simulink model "simli"  (R2023b)
settings: Solver=VariableStepAuto  StartTime=0.0  StopTime=10  RelTol=1e-3
undefined symbols (not defined in the file or in its folder): c_f, C_hv_km, Cagg, Cbase1v, Cbase_hv, Cbase_mv, delta_vsc_0, G_dc_denom, G_dc_num, H_gen, H_vsm, i_d_vsc, i_q_vsc, Ibase_hv, Ibase_mv, k_d_vsm, k_p_p_vsm, k_p_q_vsm, k_vc, ki, ki_q, kp, L_comp, l_f, l_grid, L_hv_km, l_t_ehvhv, l_t_hvmv, l_t_mvlv, Lagg, Lbase_hv, Lbase_mv, length_export, M_gr_denom, M_gr_num, mppt_gain, omega_nom, omega_WTR_0, omega_WTR_n, P_aero_0, P_meas, phase_shift_test_state, phase_shifts, pie_export, Q_meas, r_cf, r_f, r_grid, R_hv_km, r_sys, r_t_ehvhv, r_t_hvmv, r_t_mvlv, Ragg, Rd, rocof_slope, Rocof_test_state, T_dc_denom, T_dc_num, Tdelay ... (+18)
libraries: slpidlib x9, spsFirstOrderFilterLib x1, simulink x1, spsSampleandHoldLib x1, spspowerguiLib x1
(part 3 of 3)

== system simli/Subsystem/WT transformer  ==
  note: Network
  note: VIRTUAL RESITANCE
  Vpcc_DQ : Inport
  "VsDQ " : Inport  Port=2
  omega_ref : Inport  Port=3
  1 : Gain  Gain=inv_Lsource
  2 : Gain  Gain=Rsource
  3 : Gain  Gain=Rsource
  4 : Gain  Gain=inv_Lsource
  7 : Gain  Gain=Lsource
  Demux1 : Demux  Outputs=2
  Demux2 : Demux  Outputs=2
  Id : Scope
  Iline_D_int : Integrator  UpperSaturationLimit=50  LowerSaturationLimit=-1000
  Iline_Q_int : Integrator  UpperSaturationLimit=50  LowerSaturationLimit=-1000
  Iq : Scope
  Mux1 : Mux  Inputs=2
  Mux4 : Mux  Inputs=2
  Product1 : Product
  Product2 : Product
  Sum1 : Sum  Inputs=|+---
  Sum8 : Sum  Inputs=|+-+-
  Iline_DQ : Outport  VectorParamsAs1DForOutWhenUnconnected=off
  wires:
  7/1 -> [wL]
  [Vpcc_Q] -> Sum1/1
  [Vpcc_D] -> Sum8/1
  Demux2/1 -> Mux4/1, [Vpcc_D]
  Demux2/2 -> Mux4/2, [Vpcc_Q]
  Sum1/1 -> 4/1
  1/1 -> Iline_D_int/1
  Iline_D_int/1 -> Product1/2, Id/1, 2/1, Mux1/1
  Iline_Q_int/1 -> Mux1/2, Iq/1, Product2/2, 3/1
  Sum8/1 -> 1/1
  2/1 -> Sum8/4
  Product2/1 -> Sum8/3
  3/1 -> Sum1/4
  4/1 -> Iline_Q_int/1
  Product1/1 -> Sum1/3
  [wL] -> Product1/1, Product2/1
  Demux1/1 -> Sum8/2
  Demux1/2 -> Sum1/2
  "VsDQ "/1 -> Demux1/1
  Vpcc_DQ/1 -> Demux2/1
  Mux1/1 -> Iline_DQ/1
  omega_ref/1 -> 7/1

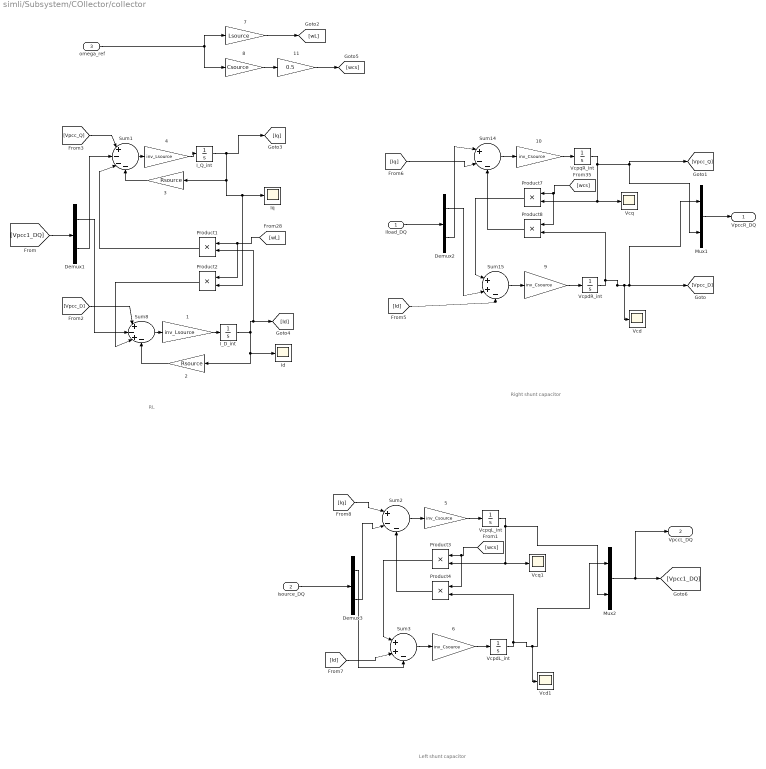
== system simli/Subsystem/COllector/collector ==
  note: RL
  note: Right shunt capacitor
  note: Left shunt capacitor
  Iload_DQ : Inport
  "Isource_DQ " : Inport  Port=2
  omega_ref : Inport  Port=3
  1 : Gain  Gain=inv_Lsource
  {5..6,9..10} (4 alike) : Gain  Gain=inv_Csource
  11 : Gain  Gain=0.5
  2 : Gain  Gain=Rsource
  3 : Gain  Gain=Rsource
  4 : Gain  Gain=inv_Lsource
  7 : Gain  Gain=Lsource
  8 : Gain  Gain=Csource
  Demux1 : Demux  Outputs=2
  Demux2 : Demux  Outputs=2
  Demux3 : Demux  Outputs=2
  I_D_int : Integrator  UpperSaturationLimit=50  LowerSaturationLimit=-1000
  I_Q_int : Integrator  UpperSaturationLimit=50  LowerSaturationLimit=-1000
  Id : Scope
  Iq : Scope
  Mux1 : Mux  Inputs=2
  Mux2 : Mux  Inputs=2
  Product{1..4,7..8} (6 alike) : Product
  Sum1 : Sum  Inputs=|+---
  Sum14 : Sum  Inputs=|+--
  Sum15 : Sum  Inputs=|++-
  Sum2 : Sum  Inputs=|+--
  Sum3 : Sum  Inputs=|++-
  Sum8 : Sum  Inputs=|+-+-
  Vcd : Scope
  Vcd1 : Scope
  VcpdL_int : Integrator  UpperSaturationLimit=50  LowerSaturationLimit=-1000
  VcpdR_int : Integrator  UpperSaturationLimit=50  LowerSaturationLimit=-1000
  VcpqL_int : Integrator  UpperSaturationLimit=50  LowerSaturationLimit=-1000
  VcpqR_int : Integrator  UpperSaturationLimit=50  LowerSaturationLimit=-1000
  Vcq : Scope
  Vcq1 : Scope
  VpccR_DQ : Outport  VectorParamsAs1DForOutWhenUnconnected=off
  VpccL_DQ : Outport  Port=2  VectorParamsAs1DForOutWhenUnconnected=off
  wires:
  Iload_DQ/1 -> Demux2/1
  Demux2/2 -> Sum14/1
  Demux2/1 -> Sum15/2
  [wL] -> Product2/1, Product1/1
  Product1/1 -> Sum1/3
  4/1 -> I_Q_int/1
  3/1 -> Sum1/4
  Product2/1 -> Sum8/3
  2/1 -> Sum8/4
  Sum8/1 -> 1/1
  I_Q_int/1 -> 3/1, Product2/2, Iq/1, [Iq]
  I_D_int/1 -> 2/1, Id/1, Product1/2, [Id]
  1/1 -> I_D_int/1
  Sum1/1 -> 4/1
  [Vpcc_D] -> Sum8/1
  [Vpcc_Q] -> Sum1/1
  omega_ref/1 -> 8/1, 7/1
  7/1 -> [wL]
  9/1 -> VcpdR_int/1
  Sum14/1 -> 10/1
  [wcs] -> Product8/1, Product7/1
  [Id] -> Sum15/3
  VcpqR_int/1 -> Mux1/2, [Vpcc_Q], Product7/2, Vcq/1
  Product7/1 -> Sum15/1
  [Iq] -> Sum14/2
  10/1 -> VcpqR_int/1
  Sum15/1 -> 9/1
  Product8/1 -> Sum14/3
  8/1 -> 11/1
  VcpdR_int/1 -> Product8/2, Mux1/1, [Vpcc_D], Vcd/1
  Mux1/1 -> VpccR_DQ/1
  Demux1/1 -> Sum8/2
  Demux1/2 -> Sum1/2
  [Vpcc1_DQ] -> Demux1/1
  VcpdL_int/1 -> Vcd1/1, Mux2/1, Product4/2
  Product4/1 -> Sum2/3
  Sum3/1 -> 6/1
  5/1 -> VcpqL_int/1
  Demux3/2 -> Sum2/2
  Product3/1 -> Sum3/1
  VcpqL_int/1 -> Vcq1/1, Product3/2, Mux2/2
  [wcs] -> Product3/1, Product4/1
  Sum2/1 -> 5/1
  6/1 -> VcpdL_int/1
  "Isource_DQ "/1 -> Demux3/1
  Demux3/1 -> Sum3/3
  [Id] -> Sum3/2
  [Iq] -> Sum2/1
  Mux2/1 -> VpccL_DQ/1, [Vpcc1_DQ]
  11/1 -> [wcs]

== system simli/Subsystem/HVAC CABLE 10 PI SEGMENTS 1/RC sys1 ==
  note: Left shunt capacitor
  note: shunt capacitor
  Iload_DQ : Inport
  "Isource_DQ " : Inport  Port=2
  omega_ref : Inport  Port=3
  1 : Gain  Gain=Rd
  10 : Gain  Gain=inv_Csource
  2 : Gain  Gain=Rd
  8 : Gain  Gain=Csource
  9 : Gain  Gain=inv_Csource
  Demux2 : Demux  Outputs=2
  Demux3 : Demux  Outputs=2
  Display1 : Display
  Display6 : Display
  Mux1 : Mux  Inputs=2
  Mux2 : Mux  Inputs=2
  Product7 : Product
  Product8 : Product
  Sum1 : Sum  Inputs=|++
  Sum14 : Sum  Inputs=|+--
  Sum15 : Sum  Inputs=|++-
  Sum2 : Sum  Inputs=|++
  Sum3 : Sum  Inputs=|+-
  Sum4 : Sum  Inputs=|+-
  Vcd : Scope
  VcpdR_int : Integrator  InitialCondition=VD0  UpperSaturationLimit=50  LowerSaturationLimit=-1000
  VcpqR_int : Integrator  InitialCondition=VQ0  UpperSaturationLimit=50  LowerSaturationLimit=-1000
  Vcq : Scope
  VpccR_DQ : Outport  VectorParamsAs1DForOutWhenUnconnected=off
  wires:
  8/1 -> [wcs], Display1/1
  Mux1/1 -> VpccR_DQ/1
  Product8/1 -> Sum14/3
  Sum15/1 -> 9/1
  10/1 -> VcpqR_int/1
  Product7/1 -> Sum15/1
  VcpqR_int/1 -> Mux2/1, Sum2/1, Product7/2, Vcq/1
  [wcs] -> Product7/1, Product8/1
  Sum14/1 -> 10/1
  9/1 -> VcpdR_int/1
  omega_ref/1 -> 8/1
  Demux2/1 -> Sum4/1, Sum15/2
  Demux2/2 -> Sum3/1, Sum14/1
  Iload_DQ/1 -> Demux2/1
  "Isource_DQ "/1 -> Demux3/1
  Demux3/2 -> Sum3/2, Sum14/2
  Demux3/1 -> Sum4/2, Sum15/3
  VcpdR_int/1 -> Mux2/2, Product8/2, Sum1/1
  Sum1/1 -> Mux1/1
  Sum2/1 -> Mux1/2
  1/1 -> Sum2/2
  2/1 -> Sum1/2
  Mux2/1 -> Display6/1
  Sum3/1 -> 1/1
  Sum4/1 -> 2/1

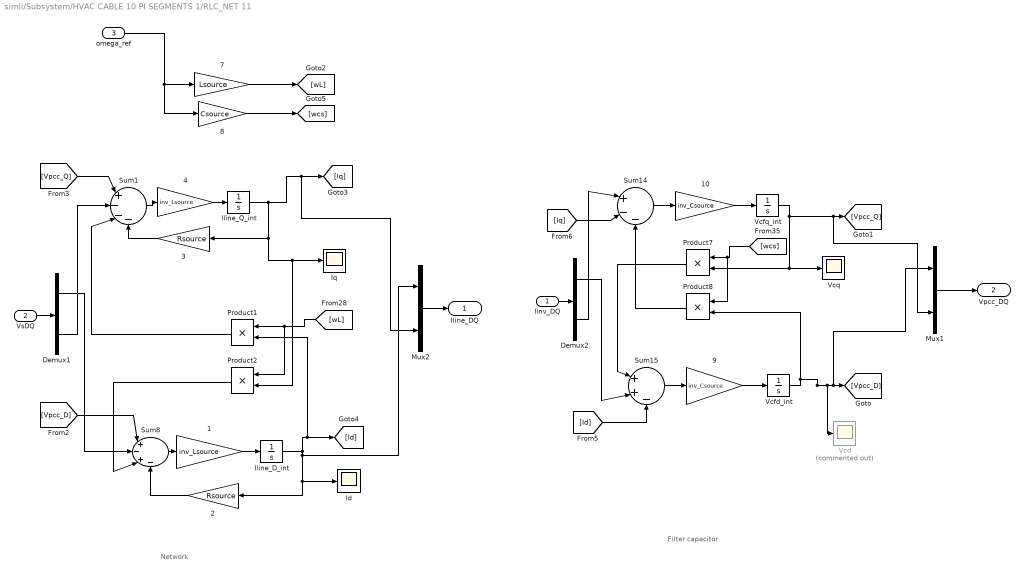
== system simli/Subsystem/HVAC CABLE 10 PI SEGMENTS 1/RLC_NET 11 ==
  note: Network
  note: Filter capacitor
  Iinv_DQ : Inport
  "VsDQ " : Inport  Port=2
  omega_ref : Inport  Port=3
  1 : Gain  Gain=inv_Lsource
  10 : Gain  Gain=inv_Csource
  2 : Gain  Gain=Rsource
  3 : Gain  Gain=Rsource
  4 : Gain  Gain=inv_Lsource
  7 : Gain  Gain=Lsource
  8 : Gain  Gain=Csource
  9 : Gain  Gain=inv_Csource
  Demux1 : Demux  Outputs=2
  Demux2 : Demux  Outputs=2
  Id : Scope
  Iline_D_int : Integrator  UpperSaturationLimit=50  LowerSaturationLimit=-1000
  Iline_Q_int : Integrator  UpperSaturationLimit=50  LowerSaturationLimit=-1000
  Iq : Scope
  Mux1 : Mux  Inputs=2
  Mux2 : Mux  Inputs=2
  Product{1..2,7..8} (4 alike) : Product
  Sum1 : Sum  Inputs=|+---
  Sum14 : Sum  Inputs=|+--
  Sum15 : Sum  Inputs=|++-
  Sum8 : Sum  Inputs=|+-+-
  Vcd : Scope  Commented=on
  Vcfd_int : Integrator  UpperSaturationLimit=50  LowerSaturationLimit=-1000
  Vcfq_int : Integrator  UpperSaturationLimit=50  LowerSaturationLimit=-1000
  Vcq : Scope
  Iline_DQ : Outport  VectorParamsAs1DForOutWhenUnconnected=off
  Vpcc_DQ : Outport  Port=2  VectorParamsAs1DForOutWhenUnconnected=off
  wires:
  Mux2/1 -> Iline_DQ/1
  Iinv_DQ/1 -> Demux2/1
  Demux2/2 -> Sum14/1
  Demux2/1 -> Sum15/2
  [wL] -> Product2/1, Product1/1
  Product1/1 -> Sum1/3
  4/1 -> Iline_Q_int/1
  3/1 -> Sum1/4
  Product2/1 -> Sum8/3
  2/1 -> Sum8/4
  Sum8/1 -> 1/1
  Iline_Q_int/1 -> 3/1, Product2/2, Iq/1, [Iq], Mux2/2
  Iline_D_int/1 -> Mux2/1, 2/1, Id/1, Product1/2, [Id]
  1/1 -> Iline_D_int/1
  Sum1/1 -> 4/1
  [Vpcc_D] -> Sum8/1
  [Vpcc_Q] -> Sum1/1
  omega_ref/1 -> 8/1, 7/1
  7/1 -> [wL]
  9/1 -> Vcfd_int/1
  Sum14/1 -> 10/1
  [wcs] -> Product8/1, Product7/1
  [Id] -> Sum15/3
  Vcfq_int/1 -> Mux1/2, [Vpcc_Q], Product7/2, Vcq/1
  Product7/1 -> Sum15/1
  [Iq] -> Sum14/2
  10/1 -> Vcfq_int/1
  Sum15/1 -> 9/1
  Product8/1 -> Sum14/3
  8/1 -> [wcs]
  Vcfd_int/1 -> Product8/2, Mux1/1, [Vpcc_D], Vcd/1
  Mux1/1 -> Vpcc_DQ/1
  Demux1/1 -> Sum8/2
  Demux1/2 -> Sum1/2
  "VsDQ "/1 -> Demux1/1

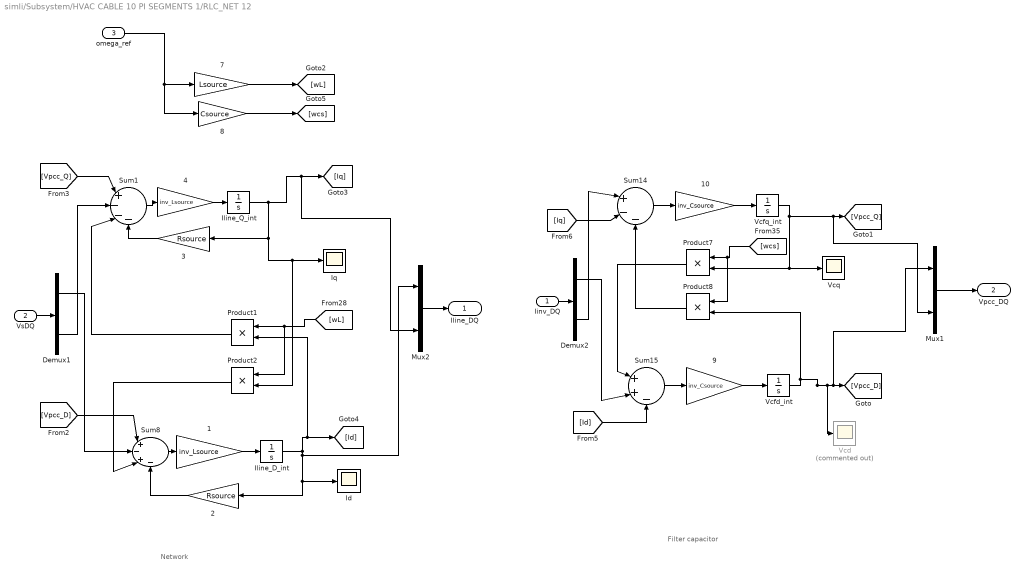
== system simli/Subsystem/HVAC CABLE 10 PI SEGMENTS 1/RLC_NET 12 ==
  note: Filter capacitor
  note: Network
  Iinv_DQ : Inport
  "VsDQ " : Inport  Port=2
  omega_ref : Inport  Port=3
  1 : Gain  Gain=inv_Lsource
  10 : Gain  Gain=inv_Csource
  2 : Gain  Gain=Rsource
  3 : Gain  Gain=Rsource
  4 : Gain  Gain=inv_Lsource
  7 : Gain  Gain=Lsource
  8 : Gain  Gain=Csource
  9 : Gain  Gain=inv_Csource
  Demux1 : Demux  Outputs=2
  Demux2 : Demux  Outputs=2
  Id : Scope
  Iline_D_int : Integrator  UpperSaturationLimit=50  LowerSaturationLimit=-1000
  Iline_Q_int : Integrator  UpperSaturationLimit=50  LowerSaturationLimit=-1000
  Iq : Scope
  Mux1 : Mux  Inputs=2
  Mux2 : Mux  Inputs=2
  Product{1..2,7..8} (4 alike) : Product
  Sum1 : Sum  Inputs=|+---
  Sum14 : Sum  Inputs=|+--
  Sum15 : Sum  Inputs=|++-
  Sum8 : Sum  Inputs=|+-+-
  Vcd : Scope  Commented=on
  Vcfd_int : Integrator  UpperSaturationLimit=50  LowerSaturationLimit=-1000
  Vcfq_int : Integrator  UpperSaturationLimit=50  LowerSaturationLimit=-1000
  Vcq : Scope
  Iline_DQ : Outport  VectorParamsAs1DForOutWhenUnconnected=off
  Vpcc_DQ : Outport  Port=2  VectorParamsAs1DForOutWhenUnconnected=off
  wires:
  "VsDQ "/1 -> Demux1/1
  Demux1/2 -> Sum1/2
  Demux1/1 -> Sum8/2
  Mux1/1 -> Vpcc_DQ/1
  Vcfd_int/1 -> Vcd/1, [Vpcc_D], Mux1/1, Product8/2
  8/1 -> [wcs]
  Product8/1 -> Sum14/3
  Sum15/1 -> 9/1
  10/1 -> Vcfq_int/1
  [Iq] -> Sum14/2
  Product7/1 -> Sum15/1
  Vcfq_int/1 -> Vcq/1, Product7/2, [Vpcc_Q], Mux1/2
  [Id] -> Sum15/3
  [wcs] -> Product7/1, Product8/1
  Sum14/1 -> 10/1
  9/1 -> Vcfd_int/1
  7/1 -> [wL]
  omega_ref/1 -> 7/1, 8/1
  [Vpcc_Q] -> Sum1/1
  [Vpcc_D] -> Sum8/1
  Sum1/1 -> 4/1
  1/1 -> Iline_D_int/1
  Iline_D_int/1 -> [Id], Product1/2, Id/1, 2/1, Mux2/1
  Iline_Q_int/1 -> Mux2/2, [Iq], Iq/1, Product2/2, 3/1
  Sum8/1 -> 1/1
  2/1 -> Sum8/4
  Product2/1 -> Sum8/3
  3/1 -> Sum1/4
  4/1 -> Iline_Q_int/1
  Product1/1 -> Sum1/3
  [wL] -> Product1/1, Product2/1
  Demux2/1 -> Sum15/2
  Demux2/2 -> Sum14/1
  Iinv_DQ/1 -> Demux2/1
  Mux2/1 -> Iline_DQ/1

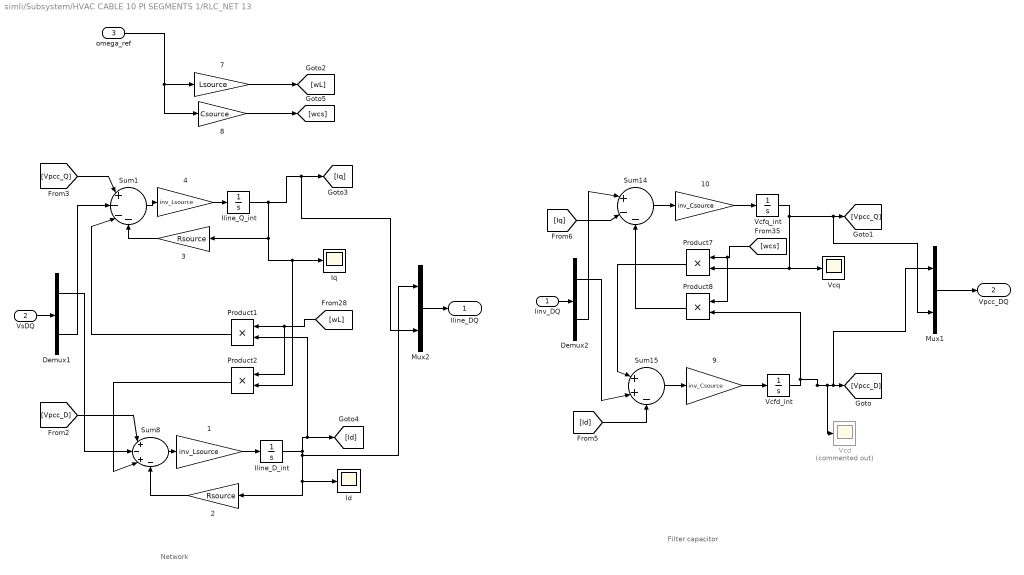
== system simli/Subsystem/HVAC CABLE 10 PI SEGMENTS 1/RLC_NET 13 ==
  note: Filter capacitor
  note: Network
  Iinv_DQ : Inport
  "VsDQ " : Inport  Port=2
  omega_ref : Inport  Port=3
  1 : Gain  Gain=inv_Lsource
  10 : Gain  Gain=inv_Csource
  2 : Gain  Gain=Rsource
  3 : Gain  Gain=Rsource
  4 : Gain  Gain=inv_Lsource
  7 : Gain  Gain=Lsource
  8 : Gain  Gain=Csource
  9 : Gain  Gain=inv_Csource
  Demux1 : Demux  Outputs=2
  Demux2 : Demux  Outputs=2
  Id : Scope
  Iline_D_int : Integrator  UpperSaturationLimit=50  LowerSaturationLimit=-1000
  Iline_Q_int : Integrator  UpperSaturationLimit=50  LowerSaturationLimit=-1000
  Iq : Scope
  Mux1 : Mux  Inputs=2
  Mux2 : Mux  Inputs=2
  Product{1..2,7..8} (4 alike) : Product
  Sum1 : Sum  Inputs=|+---
  Sum14 : Sum  Inputs=|+--
  Sum15 : Sum  Inputs=|++-
  Sum8 : Sum  Inputs=|+-+-
  Vcd : Scope  Commented=on
  Vcfd_int : Integrator  UpperSaturationLimit=50  LowerSaturationLimit=-1000
  Vcfq_int : Integrator  UpperSaturationLimit=50  LowerSaturationLimit=-1000
  Vcq : Scope
  Iline_DQ : Outport  VectorParamsAs1DForOutWhenUnconnected=off
  Vpcc_DQ : Outport  Port=2  VectorParamsAs1DForOutWhenUnconnected=off
  wires:
  "VsDQ "/1 -> Demux1/1
  Demux1/2 -> Sum1/2
  Demux1/1 -> Sum8/2
  Mux1/1 -> Vpcc_DQ/1
  Vcfd_int/1 -> Vcd/1, [Vpcc_D], Mux1/1, Product8/2
  8/1 -> [wcs]
  Product8/1 -> Sum14/3
  Sum15/1 -> 9/1
  10/1 -> Vcfq_int/1
  [Iq] -> Sum14/2
  Product7/1 -> Sum15/1
  Vcfq_int/1 -> Vcq/1, Product7/2, [Vpcc_Q], Mux1/2
  [Id] -> Sum15/3
  [wcs] -> Product7/1, Product8/1
  Sum14/1 -> 10/1
  9/1 -> Vcfd_int/1
  7/1 -> [wL]
  omega_ref/1 -> 7/1, 8/1
  [Vpcc_Q] -> Sum1/1
  [Vpcc_D] -> Sum8/1
  Sum1/1 -> 4/1
  1/1 -> Iline_D_int/1
  Iline_D_int/1 -> [Id], Product1/2, Id/1, 2/1, Mux2/1
  Iline_Q_int/1 -> Mux2/2, [Iq], Iq/1, Product2/2, 3/1
  Sum8/1 -> 1/1
  2/1 -> Sum8/4
  Product2/1 -> Sum8/3
  3/1 -> Sum1/4
  4/1 -> Iline_Q_int/1
  Product1/1 -> Sum1/3
  [wL] -> Product1/1, Product2/1
  Demux2/1 -> Sum15/2
  Demux2/2 -> Sum14/1
  Iinv_DQ/1 -> Demux2/1
  Mux2/1 -> Iline_DQ/1

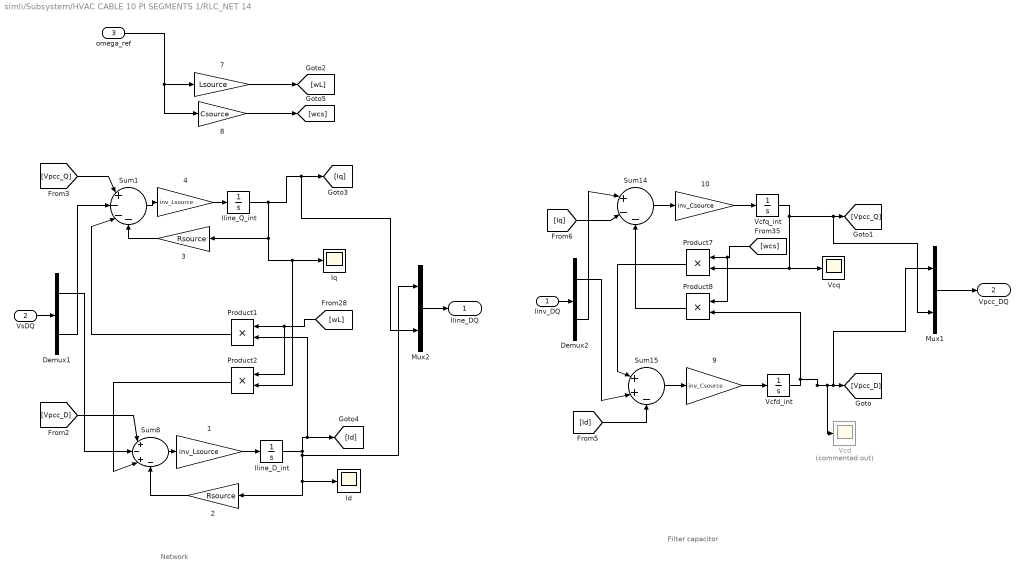
== system simli/Subsystem/HVAC CABLE 10 PI SEGMENTS 1/RLC_NET 14 ==
  note: Network
  note: Filter capacitor
  Iinv_DQ : Inport
  "VsDQ " : Inport  Port=2
  omega_ref : Inport  Port=3
  1 : Gain  Gain=inv_Lsource
  10 : Gain  Gain=inv_Csource
  2 : Gain  Gain=Rsource
  3 : Gain  Gain=Rsource
  4 : Gain  Gain=inv_Lsource
  7 : Gain  Gain=Lsource
  8 : Gain  Gain=Csource
  9 : Gain  Gain=inv_Csource
  Demux1 : Demux  Outputs=2
  Demux2 : Demux  Outputs=2
  Id : Scope
  Iline_D_int : Integrator  UpperSaturationLimit=50  LowerSaturationLimit=-1000
  Iline_Q_int : Integrator  UpperSaturationLimit=50  LowerSaturationLimit=-1000
  Iq : Scope
  Mux1 : Mux  Inputs=2
  Mux2 : Mux  Inputs=2
  Product{1..2,7..8} (4 alike) : Product
  Sum1 : Sum  Inputs=|+---
  Sum14 : Sum  Inputs=|+--
  Sum15 : Sum  Inputs=|++-
  Sum8 : Sum  Inputs=|+-+-
  Vcd : Scope  Commented=on
  Vcfd_int : Integrator  UpperSaturationLimit=50  LowerSaturationLimit=-1000
  Vcfq_int : Integrator  UpperSaturationLimit=50  LowerSaturationLimit=-1000
  Vcq : Scope
  Iline_DQ : Outport  VectorParamsAs1DForOutWhenUnconnected=off
  Vpcc_DQ : Outport  Port=2  VectorParamsAs1DForOutWhenUnconnected=off
  wires:
  Mux2/1 -> Iline_DQ/1
  Iinv_DQ/1 -> Demux2/1
  Demux2/2 -> Sum14/1
  Demux2/1 -> Sum15/2
  [wL] -> Product2/1, Product1/1
  Product1/1 -> Sum1/3
  4/1 -> Iline_Q_int/1
  3/1 -> Sum1/4
  Product2/1 -> Sum8/3
  2/1 -> Sum8/4
  Sum8/1 -> 1/1
  Iline_Q_int/1 -> 3/1, Product2/2, Iq/1, [Iq], Mux2/2
  Iline_D_int/1 -> Mux2/1, 2/1, Id/1, Product1/2, [Id]
  1/1 -> Iline_D_int/1
  Sum1/1 -> 4/1
  [Vpcc_D] -> Sum8/1
  [Vpcc_Q] -> Sum1/1
  omega_ref/1 -> 8/1, 7/1
  7/1 -> [wL]
  9/1 -> Vcfd_int/1
  Sum14/1 -> 10/1
  [wcs] -> Product8/1, Product7/1
  [Id] -> Sum15/3
  Vcfq_int/1 -> Mux1/2, [Vpcc_Q], Product7/2, Vcq/1
  Product7/1 -> Sum15/1
  [Iq] -> Sum14/2
  10/1 -> Vcfq_int/1
  Sum15/1 -> 9/1
  Product8/1 -> Sum14/3
  8/1 -> [wcs]
  Vcfd_int/1 -> Product8/2, Mux1/1, [Vpcc_D], Vcd/1
  Mux1/1 -> Vpcc_DQ/1
  Demux1/1 -> Sum8/2
  Demux1/2 -> Sum1/2
  "VsDQ "/1 -> Demux1/1

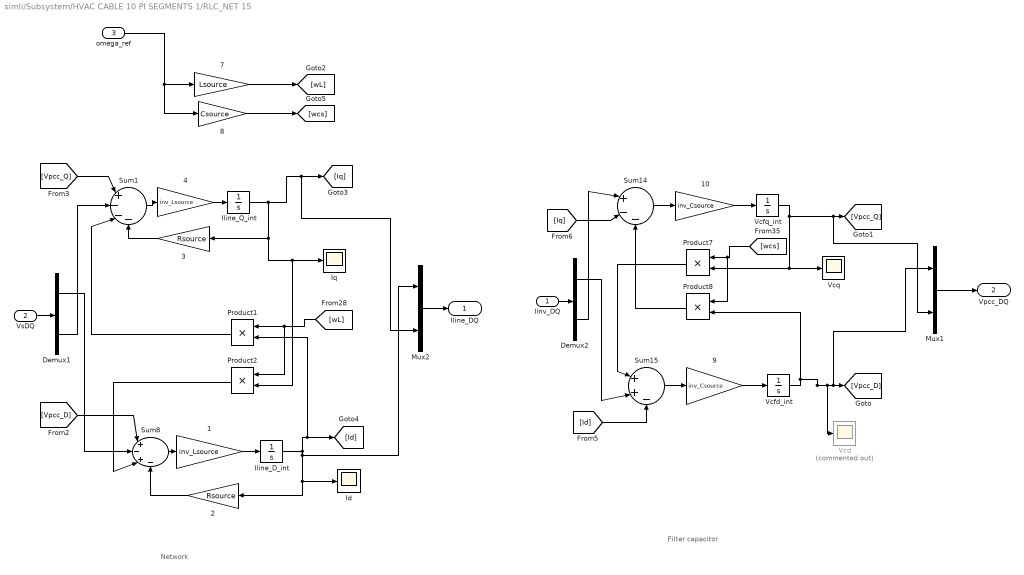
== system simli/Subsystem/HVAC CABLE 10 PI SEGMENTS 1/RLC_NET 15 ==
  note: Filter capacitor
  note: Network
  Iinv_DQ : Inport
  "VsDQ " : Inport  Port=2
  omega_ref : Inport  Port=3
  1 : Gain  Gain=inv_Lsource
  10 : Gain  Gain=inv_Csource
  2 : Gain  Gain=Rsource
  3 : Gain  Gain=Rsource
  4 : Gain  Gain=inv_Lsource
  7 : Gain  Gain=Lsource
  8 : Gain  Gain=Csource
  9 : Gain  Gain=inv_Csource
  Demux1 : Demux  Outputs=2
  Demux2 : Demux  Outputs=2
  Id : Scope
  Iline_D_int : Integrator  UpperSaturationLimit=50  LowerSaturationLimit=-1000
  Iline_Q_int : Integrator  UpperSaturationLimit=50  LowerSaturationLimit=-1000
  Iq : Scope
  Mux1 : Mux  Inputs=2
  Mux2 : Mux  Inputs=2
  Product{1..2,7..8} (4 alike) : Product
  Sum1 : Sum  Inputs=|+---
  Sum14 : Sum  Inputs=|+--
  Sum15 : Sum  Inputs=|++-
  Sum8 : Sum  Inputs=|+-+-
  Vcd : Scope  Commented=on
  Vcfd_int : Integrator  UpperSaturationLimit=50  LowerSaturationLimit=-1000
  Vcfq_int : Integrator  UpperSaturationLimit=50  LowerSaturationLimit=-1000
  Vcq : Scope
  Iline_DQ : Outport  VectorParamsAs1DForOutWhenUnconnected=off
  Vpcc_DQ : Outport  Port=2  VectorParamsAs1DForOutWhenUnconnected=off
  wires:
  "VsDQ "/1 -> Demux1/1
  Demux1/2 -> Sum1/2
  Demux1/1 -> Sum8/2
  Mux1/1 -> Vpcc_DQ/1
  Vcfd_int/1 -> Vcd/1, [Vpcc_D], Mux1/1, Product8/2
  8/1 -> [wcs]
  Product8/1 -> Sum14/3
  Sum15/1 -> 9/1
  10/1 -> Vcfq_int/1
  [Iq] -> Sum14/2
  Product7/1 -> Sum15/1
  Vcfq_int/1 -> Vcq/1, Product7/2, [Vpcc_Q], Mux1/2
  [Id] -> Sum15/3
  [wcs] -> Product7/1, Product8/1
  Sum14/1 -> 10/1
  9/1 -> Vcfd_int/1
  7/1 -> [wL]
  omega_ref/1 -> 7/1, 8/1
  [Vpcc_Q] -> Sum1/1
  [Vpcc_D] -> Sum8/1
  Sum1/1 -> 4/1
  1/1 -> Iline_D_int/1
  Iline_D_int/1 -> [Id], Product1/2, Id/1, 2/1, Mux2/1
  Iline_Q_int/1 -> Mux2/2, [Iq], Iq/1, Product2/2, 3/1
  Sum8/1 -> 1/1
  2/1 -> Sum8/4
  Product2/1 -> Sum8/3
  3/1 -> Sum1/4
  4/1 -> Iline_Q_int/1
  Product1/1 -> Sum1/3
  [wL] -> Product1/1, Product2/1
  Demux2/1 -> Sum15/2
  Demux2/2 -> Sum14/1
  Iinv_DQ/1 -> Demux2/1
  Mux2/1 -> Iline_DQ/1

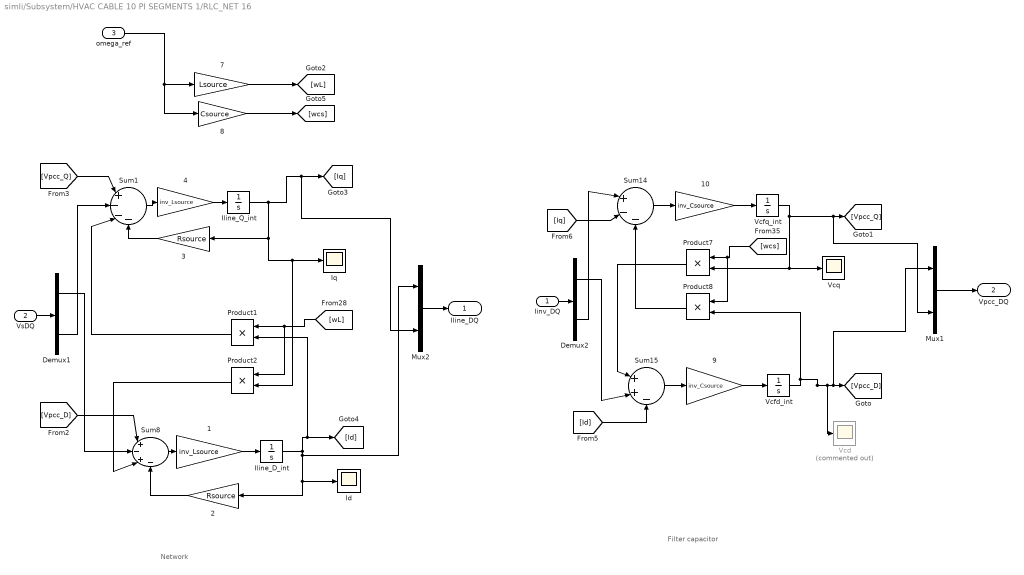
== system simli/Subsystem/HVAC CABLE 10 PI SEGMENTS 1/RLC_NET 16 ==
  note: Filter capacitor
  note: Network
  Iinv_DQ : Inport
  "VsDQ " : Inport  Port=2
  omega_ref : Inport  Port=3
  1 : Gain  Gain=inv_Lsource
  10 : Gain  Gain=inv_Csource
  2 : Gain  Gain=Rsource
  3 : Gain  Gain=Rsource
  4 : Gain  Gain=inv_Lsource
  7 : Gain  Gain=Lsource
  8 : Gain  Gain=Csource
  9 : Gain  Gain=inv_Csource
  Demux1 : Demux  Outputs=2
  Demux2 : Demux  Outputs=2
  Id : Scope
  Iline_D_int : Integrator  UpperSaturationLimit=50  LowerSaturationLimit=-1000
  Iline_Q_int : Integrator  UpperSaturationLimit=50  LowerSaturationLimit=-1000
  Iq : Scope
  Mux1 : Mux  Inputs=2
  Mux2 : Mux  Inputs=2
  Product{1..2,7..8} (4 alike) : Product
  Sum1 : Sum  Inputs=|+---
  Sum14 : Sum  Inputs=|+--
  Sum15 : Sum  Inputs=|++-
  Sum8 : Sum  Inputs=|+-+-
  Vcd : Scope  Commented=on
  Vcfd_int : Integrator  UpperSaturationLimit=50  LowerSaturationLimit=-1000
  Vcfq_int : Integrator  UpperSaturationLimit=50  LowerSaturationLimit=-1000
  Vcq : Scope
  Iline_DQ : Outport  VectorParamsAs1DForOutWhenUnconnected=off
  Vpcc_DQ : Outport  Port=2  VectorParamsAs1DForOutWhenUnconnected=off
  wires:
  "VsDQ "/1 -> Demux1/1
  Demux1/2 -> Sum1/2
  Demux1/1 -> Sum8/2
  Mux1/1 -> Vpcc_DQ/1
  Vcfd_int/1 -> Vcd/1, [Vpcc_D], Mux1/1, Product8/2
  8/1 -> [wcs]
  Product8/1 -> Sum14/3
  Sum15/1 -> 9/1
  10/1 -> Vcfq_int/1
  [Iq] -> Sum14/2
  Product7/1 -> Sum15/1
  Vcfq_int/1 -> Vcq/1, Product7/2, [Vpcc_Q], Mux1/2
  [Id] -> Sum15/3
  [wcs] -> Product7/1, Product8/1
  Sum14/1 -> 10/1
  9/1 -> Vcfd_int/1
  7/1 -> [wL]
  omega_ref/1 -> 7/1, 8/1
  [Vpcc_Q] -> Sum1/1
  [Vpcc_D] -> Sum8/1
  Sum1/1 -> 4/1
  1/1 -> Iline_D_int/1
  Iline_D_int/1 -> [Id], Product1/2, Id/1, 2/1, Mux2/1
  Iline_Q_int/1 -> Mux2/2, [Iq], Iq/1, Product2/2, 3/1
  Sum8/1 -> 1/1
  2/1 -> Sum8/4
  Product2/1 -> Sum8/3
  3/1 -> Sum1/4
  4/1 -> Iline_Q_int/1
  Product1/1 -> Sum1/3
  [wL] -> Product1/1, Product2/1
  Demux2/1 -> Sum15/2
  Demux2/2 -> Sum14/1
  Iinv_DQ/1 -> Demux2/1
  Mux2/1 -> Iline_DQ/1

== system simli/Subsystem/HVAC CABLE 10 PI SEGMENTS 1/RLC_NET 17 ==
  note: Network
  note: Filter capacitor
  Iinv_DQ : Inport
  "VsDQ " : Inport  Port=2
  omega_ref : Inport  Port=3
  1 : Gain  Gain=inv_Lsource
  10 : Gain  Gain=inv_Csource
  2 : Gain  Gain=Rsource
  3 : Gain  Gain=Rsource
  4 : Gain  Gain=inv_Lsource
  7 : Gain  Gain=Lsource
  8 : Gain  Gain=Csource
  9 : Gain  Gain=inv_Csource
  Demux1 : Demux  Outputs=2
  Demux2 : Demux  Outputs=2
  Id : Scope
  Iline_D_int : Integrator  UpperSaturationLimit=50  LowerSaturationLimit=-1000
  Iline_Q_int : Integrator  UpperSaturationLimit=50  LowerSaturationLimit=-1000
  Iq : Scope
  Mux1 : Mux  Inputs=2
  Mux2 : Mux  Inputs=2
  Product{1..2,7..8} (4 alike) : Product
  Sum1 : Sum  Inputs=|+---
  Sum14 : Sum  Inputs=|+--
  Sum15 : Sum  Inputs=|++-
  Sum8 : Sum  Inputs=|+-+-
  Vcd : Scope  Commented=on
  Vcfd_int : Integrator  UpperSaturationLimit=50  LowerSaturationLimit=-1000
  Vcfq_int : Integrator  UpperSaturationLimit=50  LowerSaturationLimit=-1000
  Vcq : Scope
  Iline_DQ : Outport  VectorParamsAs1DForOutWhenUnconnected=off
  Vpcc_DQ : Outport  Port=2  VectorParamsAs1DForOutWhenUnconnected=off
  wires:
  Mux2/1 -> Iline_DQ/1
  Iinv_DQ/1 -> Demux2/1
  Demux2/2 -> Sum14/1
  Demux2/1 -> Sum15/2
  [wL] -> Product2/1, Product1/1
  Product1/1 -> Sum1/3
  4/1 -> Iline_Q_int/1
  3/1 -> Sum1/4
  Product2/1 -> Sum8/3
  2/1 -> Sum8/4
  Sum8/1 -> 1/1
  Iline_Q_int/1 -> 3/1, Product2/2, Iq/1, [Iq], Mux2/2
  Iline_D_int/1 -> Mux2/1, 2/1, Id/1, Product1/2, [Id]
  1/1 -> Iline_D_int/1
  Sum1/1 -> 4/1
  [Vpcc_D] -> Sum8/1
  [Vpcc_Q] -> Sum1/1
  omega_ref/1 -> 8/1, 7/1
  7/1 -> [wL]
  9/1 -> Vcfd_int/1
  Sum14/1 -> 10/1
  [wcs] -> Product8/1, Product7/1
  [Id] -> Sum15/3
  Vcfq_int/1 -> Mux1/2, [Vpcc_Q], Product7/2, Vcq/1
  Product7/1 -> Sum15/1
  [Iq] -> Sum14/2
  10/1 -> Vcfq_int/1
  Sum15/1 -> 9/1
  Product8/1 -> Sum14/3
  8/1 -> [wcs]
  Vcfd_int/1 -> Product8/2, Mux1/1, [Vpcc_D], Vcd/1
  Mux1/1 -> Vpcc_DQ/1
  Demux1/1 -> Sum8/2
  Demux1/2 -> Sum1/2
  "VsDQ "/1 -> Demux1/1

== system simli/Subsystem/HVAC CABLE 10 PI SEGMENTS 1/RLC_NET 18 ==
  note: Network
  note: Filter capacitor
  Iinv_DQ : Inport
  "VsDQ " : Inport  Port=2
  omega_ref : Inport  Port=3
  1 : Gain  Gain=inv_Lsource
  10 : Gain  Gain=inv_Csource
  2 : Gain  Gain=Rsource
  3 : Gain  Gain=Rsource
  4 : Gain  Gain=inv_Lsource
  7 : Gain  Gain=Lsource
  8 : Gain  Gain=Csource
  9 : Gain  Gain=inv_Csource
  Demux1 : Demux  Outputs=2
  Demux2 : Demux  Outputs=2
  Id : Scope
  Iline_D_int : Integrator  UpperSaturationLimit=50  LowerSaturationLimit=-1000
  Iline_Q_int : Integrator  UpperSaturationLimit=50  LowerSaturationLimit=-1000
  Iq : Scope
  Mux1 : Mux  Inputs=2
  Mux2 : Mux  Inputs=2
  Product{1..2,7..8} (4 alike) : Product
  Sum1 : Sum  Inputs=|+---
  Sum14 : Sum  Inputs=|+--
  Sum15 : Sum  Inputs=|++-
  Sum8 : Sum  Inputs=|+-+-
  Vcd : Scope  Commented=on
  Vcfd_int : Integrator  UpperSaturationLimit=50  LowerSaturationLimit=-1000
  Vcfq_int : Integrator  UpperSaturationLimit=50  LowerSaturationLimit=-1000
  Vcq : Scope
  Iline_DQ : Outport  VectorParamsAs1DForOutWhenUnconnected=off
  Vpcc_DQ : Outport  Port=2  VectorParamsAs1DForOutWhenUnconnected=off
  wires:
  Mux2/1 -> Iline_DQ/1
  Iinv_DQ/1 -> Demux2/1
  Demux2/2 -> Sum14/1
  Demux2/1 -> Sum15/2
  [wL] -> Product2/1, Product1/1
  Product1/1 -> Sum1/3
  4/1 -> Iline_Q_int/1
  3/1 -> Sum1/4
  Product2/1 -> Sum8/3
  2/1 -> Sum8/4
  Sum8/1 -> 1/1
  Iline_Q_int/1 -> 3/1, Product2/2, Iq/1, [Iq], Mux2/2
  Iline_D_int/1 -> Mux2/1, 2/1, Id/1, Product1/2, [Id]
  1/1 -> Iline_D_int/1
  Sum1/1 -> 4/1
  [Vpcc_D] -> Sum8/1
  [Vpcc_Q] -> Sum1/1
  omega_ref/1 -> 8/1, 7/1
  7/1 -> [wL]
  9/1 -> Vcfd_int/1
  Sum14/1 -> 10/1
  [wcs] -> Product8/1, Product7/1
  [Id] -> Sum15/3
  Vcfq_int/1 -> Mux1/2, [Vpcc_Q], Product7/2, Vcq/1
  Product7/1 -> Sum15/1
  [Iq] -> Sum14/2
  10/1 -> Vcfq_int/1
  Sum15/1 -> 9/1
  Product8/1 -> Sum14/3
  8/1 -> [wcs]
  Vcfd_int/1 -> Product8/2, Mux1/1, [Vpcc_D], Vcd/1
  Mux1/1 -> Vpcc_DQ/1
  Demux1/1 -> Sum8/2
  Demux1/2 -> Sum1/2
  "VsDQ "/1 -> Demux1/1

== system simli/Subsystem/HVAC CABLE 10 PI SEGMENTS 1/RLC_NET 19 ==
  note: Filter capacitor
  note: Network
  Iinv_DQ : Inport
  "VsDQ " : Inport  Port=2
  omega_ref : Inport  Port=3
  1 : Gain  Gain=inv_Lsource
  10 : Gain  Gain=inv_Csource
  2 : Gain  Gain=Rsource
  3 : Gain  Gain=Rsource
  4 : Gain  Gain=inv_Lsource
  7 : Gain  Gain=Lsource
  8 : Gain  Gain=Csource
  9 : Gain  Gain=inv_Csource
  Demux1 : Demux  Outputs=2
  Demux2 : Demux  Outputs=2
  Id : Scope
  Iline_D_int : Integrator  UpperSaturationLimit=50  LowerSaturationLimit=-1000
  Iline_Q_int : Integrator  UpperSaturationLimit=50  LowerSaturationLimit=-1000
  Iq : Scope
  Mux1 : Mux  Inputs=2
  Mux2 : Mux  Inputs=2
  Product{1..2,7..8} (4 alike) : Product
  Sum1 : Sum  Inputs=|+---
  Sum14 : Sum  Inputs=|+--
  Sum15 : Sum  Inputs=|++-
  Sum8 : Sum  Inputs=|+-+-
  Vcd : Scope  Commented=on
  Vcfd_int : Integrator  UpperSaturationLimit=50  LowerSaturationLimit=-1000
  Vcfq_int : Integrator  UpperSaturationLimit=50  LowerSaturationLimit=-1000
  Vcq : Scope
  Iline_DQ : Outport  VectorParamsAs1DForOutWhenUnconnected=off
  Vpcc_DQ : Outport  Port=2  VectorParamsAs1DForOutWhenUnconnected=off
  wires:
  "VsDQ "/1 -> Demux1/1
  Demux1/2 -> Sum1/2
  Demux1/1 -> Sum8/2
  Mux1/1 -> Vpcc_DQ/1
  Vcfd_int/1 -> Vcd/1, [Vpcc_D], Mux1/1, Product8/2
  8/1 -> [wcs]
  Product8/1 -> Sum14/3
  Sum15/1 -> 9/1
  10/1 -> Vcfq_int/1
  [Iq] -> Sum14/2
  Product7/1 -> Sum15/1
  Vcfq_int/1 -> Vcq/1, Product7/2, [Vpcc_Q], Mux1/2
  [Id] -> Sum15/3
  [wcs] -> Product7/1, Product8/1
  Sum14/1 -> 10/1
  9/1 -> Vcfd_int/1
  7/1 -> [wL]
  omega_ref/1 -> 7/1, 8/1
  [Vpcc_Q] -> Sum1/1
  [Vpcc_D] -> Sum8/1
  Sum1/1 -> 4/1
  1/1 -> Iline_D_int/1
  Iline_D_int/1 -> [Id], Product1/2, Id/1, 2/1, Mux2/1
  Iline_Q_int/1 -> Mux2/2, [Iq], Iq/1, Product2/2, 3/1
  Sum8/1 -> 1/1
  2/1 -> Sum8/4
  Product2/1 -> Sum8/3
  3/1 -> Sum1/4
  4/1 -> Iline_Q_int/1
  Product1/1 -> Sum1/3
  [wL] -> Product1/1, Product2/1
  Demux2/1 -> Sum15/2
  Demux2/2 -> Sum14/1
  Iinv_DQ/1 -> Demux2/1
  Mux2/1 -> Iline_DQ/1

== system simli/Subsystem/HVAC CABLE 10 PI SEGMENTS 1/RLC_NET 20 ==
  note: Network
  note: Filter capacitor
  Iinv_DQ : Inport
  "VsDQ " : Inport  Port=2
  omega_ref : Inport  Port=3
  1 : Gain  Gain=inv_Lsource
  10 : Gain  Gain=inv_Csource
  2 : Gain  Gain=Rsource
  3 : Gain  Gain=Rsource
  4 : Gain  Gain=inv_Lsource
  7 : Gain  Gain=Lsource
  8 : Gain  Gain=Csource
  9 : Gain  Gain=inv_Csource
  Demux1 : Demux  Outputs=2
  Demux2 : Demux  Outputs=2
  Id : Scope
  Iline_D_int : Integrator  UpperSaturationLimit=50  LowerSaturationLimit=-1000
  Iline_Q_int : Integrator  UpperSaturationLimit=50  LowerSaturationLimit=-1000
  Iq : Scope
  Mux1 : Mux  Inputs=2
  Mux2 : Mux  Inputs=2
  Product{1..2,7..8} (4 alike) : Product
  Sum1 : Sum  Inputs=|+---
  Sum14 : Sum  Inputs=|+--
  Sum15 : Sum  Inputs=|++-
  Sum8 : Sum  Inputs=|+-+-
  Vcd : Scope  Commented=on
  Vcfd_int : Integrator  UpperSaturationLimit=50  LowerSaturationLimit=-1000
  Vcfq_int : Integrator  UpperSaturationLimit=50  LowerSaturationLimit=-1000
  Vcq : Scope
  Iline_DQ : Outport  VectorParamsAs1DForOutWhenUnconnected=off
  Vpcc_DQ : Outport  Port=2  VectorParamsAs1DForOutWhenUnconnected=off
  wires:
  Mux2/1 -> Iline_DQ/1
  Iinv_DQ/1 -> Demux2/1
  Demux2/2 -> Sum14/1
  Demux2/1 -> Sum15/2
  [wL] -> Product2/1, Product1/1
  Product1/1 -> Sum1/3
  4/1 -> Iline_Q_int/1
  3/1 -> Sum1/4
  Product2/1 -> Sum8/3
  2/1 -> Sum8/4
  Sum8/1 -> 1/1
  Iline_Q_int/1 -> 3/1, Product2/2, Iq/1, [Iq], Mux2/2
  Iline_D_int/1 -> Mux2/1, 2/1, Id/1, Product1/2, [Id]
  1/1 -> Iline_D_int/1
  Sum1/1 -> 4/1
  [Vpcc_D] -> Sum8/1
  [Vpcc_Q] -> Sum1/1
  omega_ref/1 -> 8/1, 7/1
  7/1 -> [wL]
  9/1 -> Vcfd_int/1
  Sum14/1 -> 10/1
  [wcs] -> Product8/1, Product7/1
  [Id] -> Sum15/3
  Vcfq_int/1 -> Mux1/2, [Vpcc_Q], Product7/2, Vcq/1
  Product7/1 -> Sum15/1
  [Iq] -> Sum14/2
  10/1 -> Vcfq_int/1
  Sum15/1 -> 9/1
  Product8/1 -> Sum14/3
  8/1 -> [wcs]
  Vcfd_int/1 -> Product8/2, Mux1/1, [Vpcc_D], Vcd/1
  Mux1/1 -> Vpcc_DQ/1
  Demux1/1 -> Sum8/2
  Demux1/2 -> Sum1/2
  "VsDQ "/1 -> Demux1/1

== system simli/Subsystem/HVAC CABLE 10 PI SEGMENTS 1/RLV_NET 1 ==
  note: Network
  note: VIRTUAL RESITANCE
  Vpcc_DQ : Inport
  omega_ref : Inport  Port=2
  1 : Gain  Gain=inv_Lsource
  2 : Gain  Gain=Rsource
  3 : Gain  Gain=Rsource
  4 : Gain  Gain=inv_Lsource
  7 : Gain  Gain=Lsource
  Demux2 : Demux  Outputs=2
  Id : Scope
  Iline_D_int : Integrator  UpperSaturationLimit=50  LowerSaturationLimit=-1000
  Iline_Q_int : Integrator  UpperSaturationLimit=50  LowerSaturationLimit=-1000
  Iq : Scope
  Mux1 : Mux  Inputs=2
  Mux4 : Mux  Inputs=2
  Product1 : Product
  Product2 : Product
  Sum1 : Sum  Inputs=|+--
  Sum8 : Sum  Inputs=|++-
  Iline_DQ : Outport  VectorParamsAs1DForOutWhenUnconnected=off
  wires:
  Mux1/1 -> Iline_DQ/1
  Product2/1 -> Sum8/2
  3/1 -> Sum1/2
  7/1 -> [wL]
  [omega_ref] -> ?
  [Vpcc_Q] -> Sum1/1
  [Vpcc_D] -> Sum8/1
  Demux2/1 -> Mux4/1, [Vpcc_D]
  Demux2/2 -> Mux4/2, [Vpcc_Q]
  Sum1/1 -> 4/1
  1/1 -> Iline_D_int/1
  Iline_D_int/1 -> Product1/2, Id/1, 2/1, Mux1/1
  Iline_Q_int/1 -> Mux1/2, Iq/1, Product2/2, 3/1
  Sum8/1 -> 1/1
  2/1 -> Sum8/3
  4/1 -> Iline_Q_int/1
  Product1/1 -> Sum1/3
  [wL] -> Product1/1, Product2/1
  Vpcc_DQ/1 -> Demux2/1
  omega_ref/1 -> 7/1

== system simli/Subsystem/HVAC CABLE 10 PI SEGMENTS 1/RLV_NET 2 ==
  note: VIRTUAL RESITANCE
  note: Network
  Vpcc_DQ : Inport
  omega_ref : Inport  Port=2
  1 : Gain  Gain=inv_Lsource
  2 : Gain  Gain=Rsource
  3 : Gain  Gain=Rsource
  4 : Gain  Gain=inv_Lsource
  7 : Gain  Gain=Lsource
  Demux2 : Demux  Outputs=2
  Id : Scope
  Iline_D_int : Integrator  UpperSaturationLimit=50  LowerSaturationLimit=-1000
  Iline_Q_int : Integrator  UpperSaturationLimit=50  LowerSaturationLimit=-1000
  Iq : Scope
  Mux1 : Mux  Inputs=2
  Mux4 : Mux  Inputs=2
  Product1 : Product
  Product2 : Product
  Sum1 : Sum  Inputs=|+--
  Sum8 : Sum  Inputs=|++-
  Iline_DQ : Outport  VectorParamsAs1DForOutWhenUnconnected=off
  wires:
  omega_ref/1 -> 7/1
  Vpcc_DQ/1 -> Demux2/1
  [wL] -> Product2/1, Product1/1
  Product1/1 -> Sum1/3
  4/1 -> Iline_Q_int/1
  2/1 -> Sum8/3
  Sum8/1 -> 1/1
  Iline_Q_int/1 -> 3/1, Product2/2, Iq/1, Mux1/2
  Iline_D_int/1 -> Mux1/1, 2/1, Id/1, Product1/2
  1/1 -> Iline_D_int/1
  Sum1/1 -> 4/1
  Demux2/2 -> [Vpcc_Q], Mux4/2
  Demux2/1 -> [Vpcc_D], Mux4/1
  [Vpcc_D] -> Sum8/1
  [Vpcc_Q] -> Sum1/1
  [omega_ref] -> ?
  7/1 -> [wL]
  3/1 -> Sum1/2
  Product2/1 -> Sum8/2
  Mux1/1 -> Iline_DQ/1
